simulink model "AVR_parameteric__"  (R2022a)
settings: Solver=VariableStepAuto  StartTime=0.0  StopTime=150  RelTol=1e-3
settings Model: Creator=asus  LastModifiedBy=asus

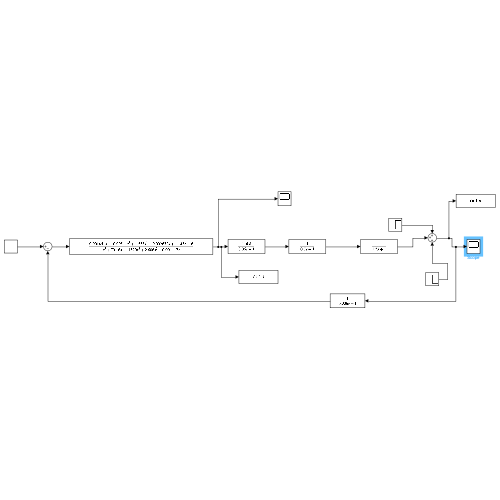
[thumbnail: Simulink's stored preview of the top-level diagram]
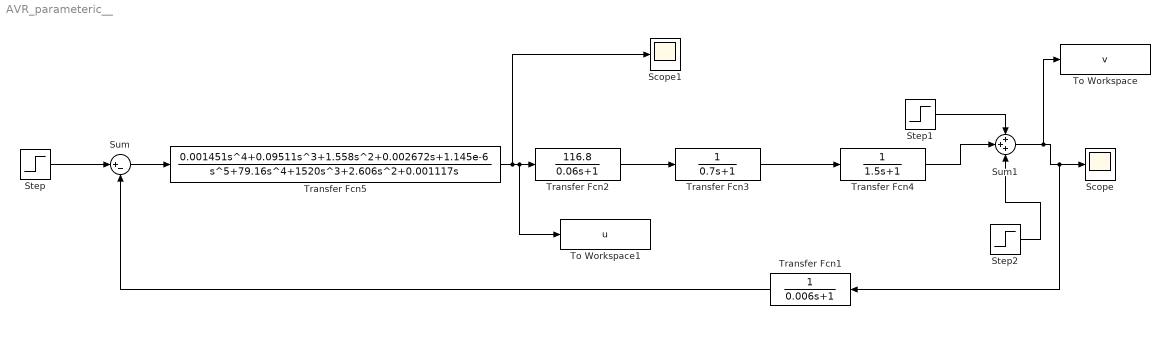
== system AVR_parameteric__ ==
  Scope : Scope
  Scope1 : Scope
  Step : Step  Time=0  SampleTime=0
  Step1 : Step  Time=50  SampleTime=0
  Step2 : Step  Time=100  After=-1  SampleTime=0
  Sum : Sum  Inputs=|+-
  Sum1 : Sum  Inputs=+++
  To Workspace : ToWorkspace  VariableName=v  SaveFormat=Timeseries  SampleTime=-1
  To Workspace1 : ToWorkspace  VariableName=u  SaveFormat=Timeseries  SampleTime=-1
  Transfer Fcn1 : TransferFcn  Denominator=[0.006 1]
  Transfer Fcn2 : TransferFcn  Numerator=[116.8]  Denominator=[0.06 1]
  Transfer Fcn3 : TransferFcn  Denominator=[0.7 1]
  Transfer Fcn4 : TransferFcn  Denominator=[1.5 1]
  Transfer Fcn5 : TransferFcn  Numerator=[0.001451 0.09511 1.558 0.002672 1.145e-6]  Denominator=[1 79.16 1520 2.606 0.001117 0]
  wires:
  Step/1 -> Sum/1
  Transfer Fcn1/1 -> Sum/2
  Step1/1 -> Sum1/1
  Sum1/1 -> To Workspace/1, Transfer Fcn1/1, Scope/1
  Step2/1 -> Sum1/3
  Transfer Fcn3/1 -> Transfer Fcn4/1
  Transfer Fcn2/1 -> Transfer Fcn3/1
  Transfer Fcn4/1 -> Sum1/2
  Sum/1 -> Transfer Fcn5/1
  Transfer Fcn5/1 -> Scope1/1, To Workspace1/1, Transfer Fcn2/1
